simulink model "exampleIAMtable"  (R2013b)
settings: Solver=ode45  StartTime=0  StopTime=300  RelTol=1e-3
undefined symbols (not defined in the file): Incidence_Angle_sun, Solar_Radiation_diffuse_surface, Solar_Radiation_direct_surface
libraries: carnot x2, simulink_extras x1, simulink x1
settings Model: Creator=drhf  LastModifiedBy=drhf
settings OptimizationCC: ExpressionDepthLimit=2147483647
settings DebuggingCC: StateNameClashWarn=warning
settings GRTTargetCC: CombineOutputUpdateFcns=off  GRTInterface=on

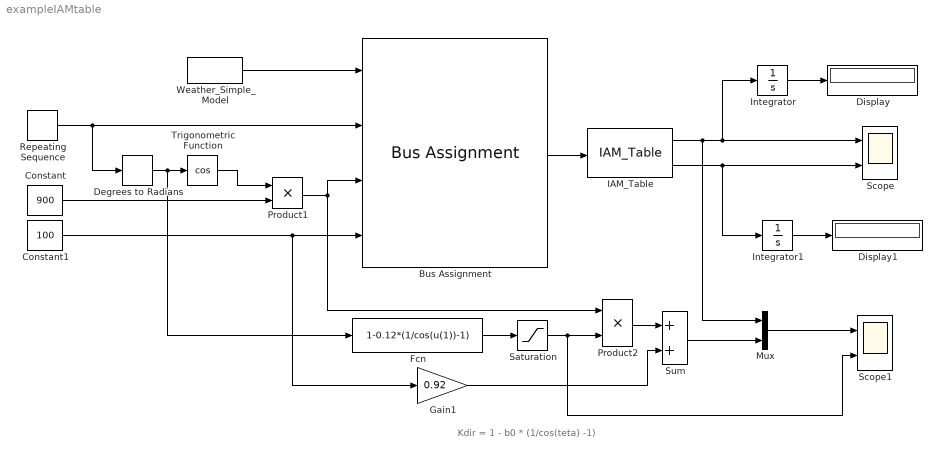
== system exampleIAMtable ==
  note: Kdir = 1 - b0 * (1/cos(teta) -1)
  Bus Assignment : BusAssignment  AssignedSignals=Incidence_Angle_sun,Solar_Radiation_direct_surface,Solar_Radiation_diffuse_surface
  Constant : Constant  Value=900
  Constant1 : Constant  Value=100
  Degrees to Radians : simulink_extras/Transformations/Degrees to Radians
  Display : Display
  Display1 : Display
  Fcn : Fcn  Expr=1-0.12*(1/cos(u(1))-1)
  Gain1 : Gain  Gain=0.92
  IAM_Table : carnot/Source/Solar_Thermal/IncidenceAngleModifier/IAM_Table  fta=1  angle=[0:5:90]  Kb="[1.0000    1.0000    0.9999    0.9996    0.9991    0.9982    0.9965  0.9935    0.9886    0.9807    0.9678    0.9473    0.9148    0.8638   0.7846    0.6644    0.4907    0.2599    0.0000]"  Kd=0.92
  Integrator : Integrator
  Integrator1 : Integrator
  Mux : Mux  Inputs=2
  Product1 : Product  RndMeth=Zero
  Product2 : Product  RndMeth=Zero
  Repeating Sequence : simulink/Sources/Repeating Sequence  rep_seq_t=[0 100]  rep_seq_y=[0 90]
  Saturation : Saturate  UpperLimit=inf  LowerLimit=0
  Scope : Scope  NumInputPorts=2
      settings: YMin=-5~-5  YMax=5~5
  Scope1 : Scope  NumInputPorts=2
      settings: YMin=-5~-5  YMax=5~5
  Sum : Sum  SaturateOnIntegerOverflow=on  InputSameDT=on  OutDataTypeStr=Inherit: Same as first input
  Trigonometric Function : Trigonometry  Operator=cos
  Weather_Simple_Model : carnot/Weather/Weather_Simple_Model  lat=60  Ibn=900  Idg=100  tamb=5  deltaTsky=-6  rh=50  precip="10e-3/24/3600           % 10 mm in 24 h"  cloud=0.125  p=1013e2  vw=1  wdir=270
  wires:
  IAM_Table/1 -> Scope/1, Integrator/1, Mux/1
  IAM_Table/2 -> Integrator1/1, Scope/2
  Integrator/1 -> Display/1
  Weather_Simple_Model/1 -> Bus Assignment/1
  Bus Assignment/1 -> IAM_Table/1
  Repeating Sequence/1 -> Bus Assignment/2, Degrees to Radians/1
  Constant/1 -> Product1/2
  Constant1/1 -> Gain1/1, Bus Assignment/4
  Product1/1 -> Product2/1, Bus Assignment/3
  Degrees to Radians/1 -> Trigonometric Function/1, Fcn/1
  Trigonometric Function/1 -> Product1/1
  Integrator1/1 -> Display1/1
  Gain1/1 -> Sum/2
  Product2/1 -> Sum/1
  Fcn/1 -> Saturation/1
  Sum/1 -> Mux/2
  Mux/1 -> Scope1/1
  Saturation/1 -> Product2/2, Scope1/2
